simulink model "ballBounce_dynamic"  (R2018b)
settings: Solver=ode23  StartTime=0.0  StopTime=25  MaxStep=0.01  RelTol=1e-3  AbsTol=1E-6  EnableMultiTasking=on
Description:
  | Bouncing Ball Model
  | 
  | This model calculates the trajectory, over time, of a ball thrown
  | upward with a velocity of 15 meters per second from a height of 10 m.
  | The model demonstrates the use of the 'ReinitDXDTwhenXreachesSaturation'
  | parameter in the Second-Order Integrator block to model this system.
  | This parameter, when set to 'on', forces a reinitialization of dx/dt
  | (velocity in the model) at the instant when x (position) reaches
  | saturation (i.e., when the ball hits the ground). The reinitialized value
  | is calculated by multiplying a coefficient of restitution times the ball
  | velocity, the instant before the ball hits the ground. The Memory block
  | in the calculation loop serves to capture the velocity of the ball just
  | before it hits the ground. The position of the ball is plotted in the
  | upper axis of the scope while the velocity of the ball is plotted in
  | the lower axis.
settings Model: Creator=The MathWorks, Inc.  LastModifiedBy=dmohtasham
settings SolverCC: AutoScaleAbsTol=off
settings DataIOCC: MaxDataPoints=7500  SaveFormat=Array  SaveOutput=off  SignalLogging=off  DSMLogging=off  SaveTime=off
settings OptimizationCC: ExpressionDepthLimit=2147483647  EfficientFloat2IntCast=on  LifeSpan=inf
settings DebuggingCC: UnderspecifiedInitializationDetection=Classic  MergeDetectMultiDrivingBlocksExec=none  IgnoredZcDiagnostic=none  FcnCallInpInsideContextMsg=warning  StateNameClashWarn=warning  SFUnexpectedBacktrackingDiag=warning  SFNoUnconditionalDefaultTransitionDiag=warning  SFExecutionAtInitializationDiag=none
settings HardwareCC: ProdBitPerPointer=32  ProdBitPerSizeT=32  ProdBitPerPtrDiffT=32  ProdLargestAtomicFloat=None  ProdIntDivRoundTo=Undefined  ProdEndianess=Unspecified  ProdWordSize=32  ProdHWDeviceType=32-bit Generic  TargetBitPerLong=64  TargetBitPerPointer=64  TargetBitPerSizeT=64  TargetBitPerPtrDiffT=64  TargetLongLongMode=on  TargetIntDivRoundTo=Zero  TargetEndianess=LittleEndian  TargetWordSize=64  TargetHWDeviceType=MATLAB Host  ProdEqTarget=off
settings ModelReferenceCC: PropagateSignalLabelsOutOfModel=off
settings SFSimCC: SimUseLocalCustomCode=off
settings RTWCC: SystemTargetFile=rsim.tlc  TemplateMakefile=rsim_default_tmf  Description=Rapid Simulation Target  RTWUseLocalCustomCode=off
settings CodeAppCC: StateflowObjectComments=on
settings TargetCC: ParMdlRefBuildCompliant=on  ConcurrentExecutionCompliant=on  MatFileLogging=on  PreserveStateflowLocalDataDimensions=off
settings ConfigComp: CovMetricSettings=dw  CovHtmlReporting=on  CovSaveCumulativeToWorkspaceVar=on  CovSaveSingleToWorkspaceVar=on  CovExternalEMLEnable=off

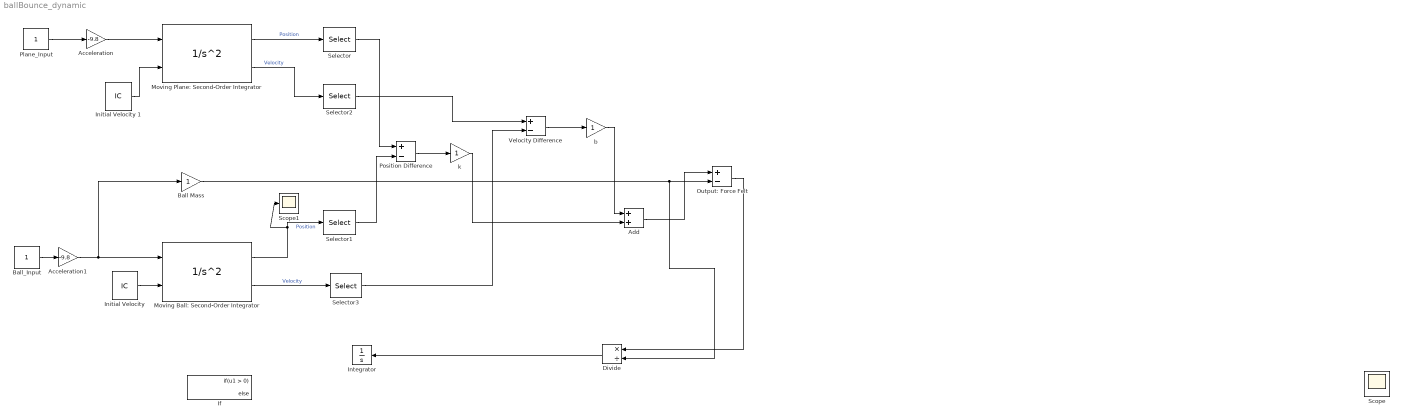
== system ballBounce_dynamic ==
  Acceleration : Gain  Gain=-9.8
  Acceleration1 : Gain  Gain=-9.8
  Add : Sum
  Ball Mass : Gain
  Ball_Input : Constant  OutDataTypeStr=double
  Divide : Product  Inputs=*/
  If : If
  "Initial Velocity " : InitialCondition  Value=-10
  Initial Velocity 1 : InitialCondition  Value=-10
  Integrator : Integrator
  Moving Ball: Second-Order Integrator : SecondOrderIntegrator  ICX=5  LimitX=on  LowerLimitX=0.0  StateNameX='Position'  ICSourceDXDT=external  StateNameDXDT='Velocity'  ReinitDXDTwhenXreachesSaturation=on
  Moving Plane: Second-Order Integrator : SecondOrderIntegrator  ICX=10.0  LimitX=on  LowerLimitX=0.0  StateNameX='Position'  ICSourceDXDT=external  StateNameDXDT='Velocity'  ReinitDXDTwhenXreachesSaturation=on
  Output: Force Felt : Sum  Inputs=+-
  Plane_Input : Constant  OutDataTypeStr=double
  "Position Difference " : Sum  Inputs=+-
  Scope1 : Scope
  Selector{,1..3} (4 alike) : Selector  NumberOfDimensions=2  InputPortWidth=3  IndexOptions=Index vector (dialog),Select all  Indices=[1 3],1  OutputSizes=1,1
  Velocity Difference : Sum  Inputs=+-
  b : Gain
  k : Gain
  Scope : Scope
  wires:
  Ball_Input/1 -> Acceleration1/1
  Moving Ball: Second-Order Integrator/1 -> Scope1/1, Selector1/1  "Position"
  Moving Ball: Second-Order Integrator/2 -> Selector3/1  "Velocity"
  "Initial Velocity "/1 -> Moving Ball: Second-Order Integrator/2
  Plane_Input/1 -> Acceleration/1
  Moving Plane: Second-Order Integrator/1 -> Selector/1  "Position"
  Moving Plane: Second-Order Integrator/2 -> Selector2/1  "Velocity"
  Selector/1 -> "Position Difference "/1
  Selector1/1 -> "Position Difference "/2
  "Position Difference "/1 -> k/1
  Selector2/1 -> Velocity Difference/1
  Selector3/1 -> Velocity Difference/2
  Velocity Difference/1 -> b/1
  k/1 -> Add/2
  b/1 -> Add/1
  Ball Mass/1 -> Divide/2, Output: Force Felt/2
  Add/1 -> Output: Force Felt/1
  Acceleration/1 -> Moving Plane: Second-Order Integrator/1
  Acceleration1/1 -> Ball Mass/1, Moving Ball: Second-Order Integrator/1
  Initial Velocity 1/1 -> Moving Plane: Second-Order Integrator/2
  Output: Force Felt/1 -> Divide/1
  Divide/1 -> Integrator/1
